simulink model "asbAUV"  (R2024b)
settings: Solver=VariableStepAuto  StartTime=0.0  StopTime=300  FixedStep=0.5  RelTol=1e-3
InitFcn:
  | mdlWks = get_param(gcs,'ModelWorkspace');
  | a = getVariable(mdlWks,'a');
  | b = getVariable(mdlWks,'b');
  | c = getVariable(mdlWks,'c');
StopFcn:
  | fTraj = findobj("Tag","asbAUVTrajectory");
  | 
  | if isempty(fTraj)
  |    fTraj = figure("Tag","asbAUVTrajectory");
  |    axes(fTraj);
  | end
  | 
  | axTraj= gca(fTraj);
  | 
  | if exist('PositionData', 'var')
  |    plot3(axTraj,PositionData(1,1),PositionData(1,2),PositionData(1,3),'r*')
  |    hold on
  |    plot3(axTraj,PositionData(:,1),PositionData(:,2),PositionData(:,3));
  |    plot3(axTraj,PositionData(end,1),PositionData(end,2),PositionData(end,3),'g*');
  | 
  |    axTraj.XLim = [0 15];
  |    axTraj.YLim = [-10 2];
  |    axTraj.ZLim = [-2 12];
  |    axTraj.XLabel.String = 'X (m)';
  |    axTraj.YLabel.String = 'Y (m)';
  |    axTraj.ZLabel.String = 'Z (m)';
  |    grid on
  |    hold off
  | 
  |    legend(axTraj,{'Start Point','Trajectory','End Point'});
  | end
model workspace (MAT data in the model file):
  a = 1
  b = 0
  c = 0
libraries: asbAUVlib x29, dspfdesign x6, slpidlib x6, shared6dof x1, aerolibasang x1, sharedutil x1, aerolibnav x1, SignalEditorBlockLib x1
(part 2 of 3)

== system asbAUV/Plant and Environment Model ==
  Thrust Control : Inport
  Combine Forces and Moments : Subsystem
  Dynamics solver : Subsystem
  Environmental Forces & Moments : Subsystem
  Propulsion Forces & Moments : Subsystem
  Outport : Outport  VectorParamsAs1DForOutWhenUnconnected=off
  wires:
  Thrust Control/1 -> Propulsion Forces & Moments/1(Thrust Control In)
  Propulsion Forces & Moments/1(Propulsion Parameters) -> Combine Forces and Moments/1(Propulsion Parameters)
  Environmental Forces & Moments/1(Environment Parameters) -> Combine Forces and Moments/2(Hydrodynamic Force)
  Combine Forces and Moments/1(Total Force) -> Dynamics solver/1(Total Force)
  Combine Forces and Moments/2(Total Moment) -> Dynamics solver/2(Total Moment)
  Dynamics solver/1(AUV Data) -> Outport/1
  Dynamics solver/2(Internal Parameters) -> Environmental Forces & Moments/1(AOA_SideSlip)

== system asbAUV/Sensor data and State Estimation ==
  AUV_Parameters : Inport
  System With Noise : Subsystem  VariantControl=c==0
  System without Noise : Subsystem  VariantControl=c==1
  Filtered Parameters : Outport  VectorParamsAs1DForOutWhenUnconnected=off

== system asbAUV/Switch Parameters ==
  Constant : Constant  Value=a
  Constant1 : Constant  Value=b
  Constant2 : Constant  Value=c
  Terminator1 : Terminator
  Terminator2 : Terminator
  Terminator3 : Terminator
  wires:
  Constant/1 -> Terminator1/1
  Constant1/1 -> Terminator2/1
  Constant2/1 -> Terminator3/1

== system asbAUV/Translation Controller ==
  Actual Parameters : Inport
  Reference Parameters : Inport  Port=2
  Position Controller : Subsystem  VariantControl=a==0
  Velocity Controller : Subsystem  VariantControl=a==1
  Thrust Control : Outport  VectorParamsAs1DForOutWhenUnconnected=off

== system asbAUV/Translational Reference ==
  Bus Creator : BusCreator  Inputs=2
  Signal Editor : SignalEditorBlockLib/Signal Editor  FileName=asbTransRefScenario.mat  ActiveScenario=asbTransrefScenario  ActiveSignal=Reference Velocity  IsBus=off  OutputBusObjectStr=Bus: BusObject  SampleTime=0  Interpolate=off  ZeroCross=off  OutputAfterFinalValue=Holding final value  Unit=inherit  PreserveSignalName=on  ApplySigPropsToAllScenarios=on  ApplySigPropsToAllSignals=off
  Reference Parameters : Outport  VectorParamsAs1DForOutWhenUnconnected=off
  wires:
  Signal Editor/1 -> Bus Creator/1  "Reference Position"
  Signal Editor/2 -> Bus Creator/2  "Reference Velocity"
  Bus Creator/1 -> Reference Parameters/1

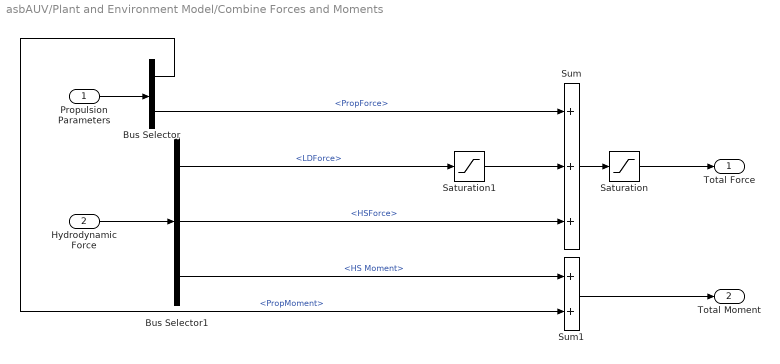
== system asbAUV/Plant and Environment Model/Combine Forces and Moments ==
  Propulsion Parameters : Inport
  Hydrodynamic Force : Inport  Port=2
  Bus Selector : BusSelector  OutputSignals=PropMoment,PropForce
  Bus Selector1 : BusSelector  OutputSignals=LDForce,HSForce,HS Moment
  Saturation : Saturate  UpperLimit=600  LowerLimit=-600
  Saturation1 : Saturate  UpperLimit=600  LowerLimit=-600
  Sum : Sum  Inputs=+++
  Sum1 : Sum
  Total Force : Outport  VectorParamsAs1DForOutWhenUnconnected=off
  Total Moment : Outport  Port=2  VectorParamsAs1DForOutWhenUnconnected=off
  wires:
  Bus Selector1/3 -> Sum1/1  "<HS Moment>"
  Bus Selector/1 -> Sum1/2  "<PropMoment>"
  Sum/1 -> Saturation/1
  Sum1/1 -> Total Moment/1
  Saturation1/1 -> Sum/2
  Saturation/1 -> Total Force/1
  Propulsion Parameters/1 -> Bus Selector/1
  Hydrodynamic Force/1 -> Bus Selector1/1
  Bus Selector/2 -> Sum/1  "<PropForce>"
  Bus Selector1/1 -> Saturation1/1  "<LDForce>"
  Bus Selector1/2 -> Sum/3  "<HSForce>"

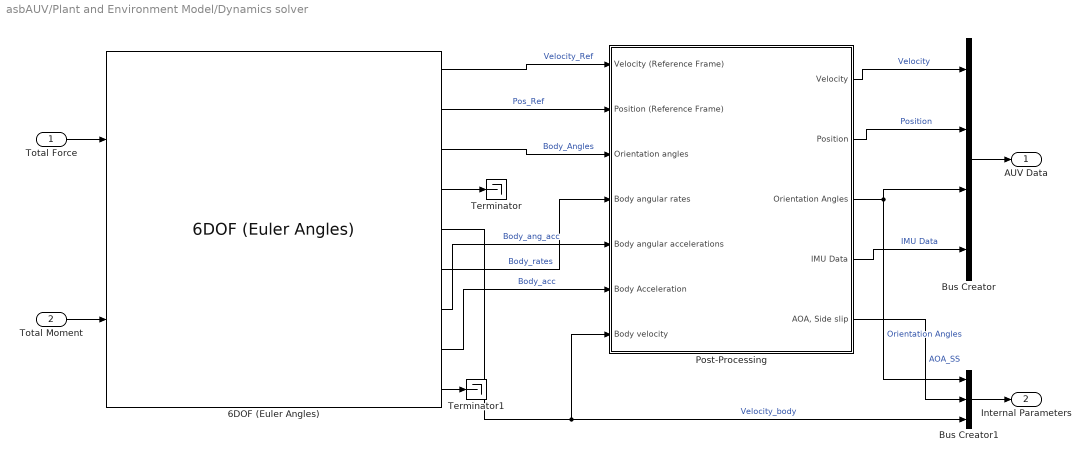
== system asbAUV/Plant and Environment Model/Dynamics solver ==
  Total Force : Inport
  Total Moment : Inport  Port=2
  6DOF (Euler Angles) : shared6dof/6DOF (Euler Angles)  units=Metric (MKS)  mtype=Fixed  rep=Euler Angles  xme_0=[0.01 .01 .01]  Vm_0=[0.01 0.01 0.001]  eul_0=[0.001 0.001 0.001]  pm_0=[0.001 0.001 0.001]  mass_0=10  mass_e=0.5  mass_f=2.0  inertia=10*eye(3)  inertia_e=eye(3)  inertia_f=2*eye(3)  k_quat=1.0  vre_flag=on  abi_flag=on  aMode=0  xme_statename=''  Vm_statename=''  eul_statename=''  quat_statename=''  pm_statename=''  mass_statename=''
  Bus Creator : BusCreator  Inputs=4
  Bus Creator1 : BusCreator  Inputs=3
  Post-Processing : Subsystem
  Terminator : Terminator
  Terminator1 : Terminator
  AUV Data : Outport  VectorParamsAs1DForOutWhenUnconnected=off
  Internal Parameters : Outport  Port=2  VectorParamsAs1DForOutWhenUnconnected=off
  wires:
  6DOF (Euler Angles)/6 -> Post-Processing/4(Body angular rates)  "Body_rates"
  Post-Processing/5("AOA, Side slip") -> Bus Creator1/2  "AOA_SS"
  6DOF (Euler Angles)/8 -> Post-Processing/6(Body Acceleration)  "Body_acc"
  Post-Processing/2(" Position") -> Bus Creator/2  "Position"
  6DOF (Euler Angles)/7 -> Post-Processing/5(Body angular accelerations)  "Body_ang_acc"
  6DOF (Euler Angles)/2 -> Post-Processing/2(Position (Reference Frame))  "Pos_Ref"
  6DOF (Euler Angles)/3 -> Post-Processing/3(Orientation angles)  "Body_Angles"
  Post-Processing/1(Velocity) -> Bus Creator/1  "Velocity"
  6DOF (Euler Angles)/1 -> Post-Processing/1(Velocity (Reference Frame))  "Velocity_Ref"
  6DOF (Euler Angles)/5 -> Bus Creator1/3, Post-Processing/7(Body velocity)  "Velocity_body"
  Post-Processing/3(Orientation Angles) -> Bus Creator/3, Bus Creator1/1  "Orientation Angles"
  Post-Processing/4(IMU Data) -> Bus Creator/4  "IMU Data"
  Total Force/1 -> 6DOF (Euler Angles)/1
  Total Moment/1 -> 6DOF (Euler Angles)/2
  Bus Creator/1 -> AUV Data/1
  Bus Creator1/1 -> Internal Parameters/1
  6DOF (Euler Angles)/4 -> Terminator/1
  6DOF (Euler Angles)/9 -> Terminator1/1

== system asbAUV/Plant and Environment Model/Environmental Forces & Moments ==
  AOA_SideSlip : Inport
  Bus Creator : BusCreator  Inputs=3
  Bus Selector : BusSelector  OutputSignals=Velocity_body,AOA_SS,Orientation Angles
  Hydrodynamic Forces : Subsystem  Variant=on
  Hydrostatic Forces : Subsystem
  Environment Parameters : Outport  VectorParamsAs1DForOutWhenUnconnected=off
  wires:
  Hydrodynamic Forces/1("Force due to Lift, Drag") -> Bus Creator/1  "LDForce"
  Hydrostatic Forces/1(Hydrostatic Force) -> Bus Creator/2  "HSForce"
  Hydrostatic Forces/2(Hydrostatic Moment) -> Bus Creator/3  "HS Moment"
  Bus Creator/1 -> Environment Parameters/1
  AOA_SideSlip/1 -> Bus Selector/1
  Bus Selector/1 -> Hydrodynamic Forces/1("Submarine Velocity (Body Axis) ")  "<Velocity_body>"
  Bus Selector/2 -> Hydrodynamic Forces/2("AOA, Side Slip")  "<AOA_SS>"
  Bus Selector/3 -> Hydrostatic Forces/1(In1)  "<Orientation Angles>"

== system asbAUV/Plant and Environment Model/Propulsion Forces & Moments ==
  Thrust Control In : Inport
  Bus Creator : BusCreator  Inputs=2
  Force and moments due to Thrust : Subsystem
  Input commands to Thrust : Subsystem
  Propulsion Parameters : Outport  VectorParamsAs1DForOutWhenUnconnected=off
  wires:
  Input commands to Thrust/1(Thrust values) -> Force and moments due to Thrust/1(Thrust Inputs)
  Thrust Control In/1 -> Input commands to Thrust/1(Thrust Control Inputs)
  Force and moments due to Thrust/1(Propulsion Force) -> Bus Creator/1  "PropForce"
  Force and moments due to Thrust/2(Propulsion Moment) -> Bus Creator/2  "PropMoment"
  Bus Creator/1 -> Propulsion Parameters/1

== system asbAUV/Sensor data and State Estimation/System With Noise ==
  AUV_Parameters : Inport
  " Sensor (IMU)" : Subsystem
  Internal filter : Subsystem
  Filtered Parameters : Outport  VectorParamsAs1DForOutWhenUnconnected=off
  wires:
  AUV_Parameters/1 -> " Sensor (IMU)"/1(IMU Inputs)
  Internal filter/1(Filtered Parameters) -> Filtered Parameters/1
  " Sensor (IMU)"/1(IMU Measurements) -> Internal filter/1(Accel)

== system asbAUV/Sensor data and State Estimation/System without Noise ==
  AUV_Parameters : Inport
  Bus Creator : BusCreator  Inputs=2
  Bus Selector : BusSelector  OutputSignals=Position,Velocity
  Gain : Gain
  Gain1 : Gain
  Filtered Parameters : Outport  VectorParamsAs1DForOutWhenUnconnected=off
  wires:
  Bus Creator/1 -> Filtered Parameters/1
  Bus Selector/2 -> Gain1/1  "<Velocity>"
  Bus Selector/1 -> Gain/1  "<Position>"
  Gain1/1 -> Bus Creator/2  "Filtered Velocity"
  Gain/1 -> Bus Creator/1  "Filtered Position"
  AUV_Parameters/1 -> Bus Selector/1

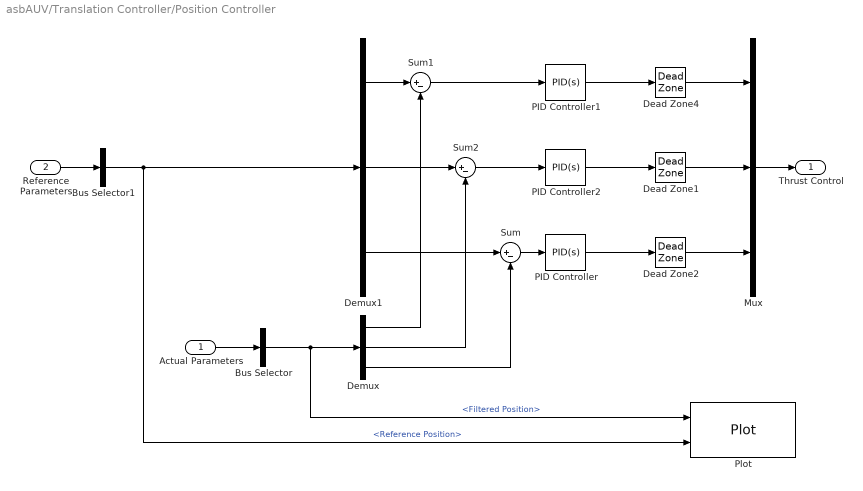
== system asbAUV/Translation Controller/Position Controller ==
  Actual Parameters : Inport
  Reference Parameters : Inport  Port=2
  Bus Selector : BusSelector  OutputSignals=Filtered Position
  Bus Selector1 : BusSelector  OutputSignals=Reference Position
  Dead Zone1 : DeadZone  LowerValue=-0.05  UpperValue=+0.05
  Dead Zone2 : DeadZone  LowerValue=-0.05  UpperValue=+0.05
  Dead Zone4 : DeadZone  LowerValue=-0.05  UpperValue=+0.05
  Demux : Demux  Outputs=3
  Demux1 : Demux  Outputs=3
  Mux : Mux  Inputs=3
  PID Controller : slpidlib/PID Controller  Controller=PID  Form=Parallel  TimeDomain=Continuous-time  UseExternalTs=off  SampleTime=-1  IntegratorMethod=Forward Euler  FilterMethod=Forward Euler  ControllerParametersSource=internal  P=-0.0440831016133051  I=-0.00046335965727533  UseKiTs=off  D=-0.931852208113014  UseExternalDerivativeSource=off  N=205.904485551143  UseFilter=on  TunerSelectOption=Transfer Function Based (PID Tuner App)  InitialConditionSource=internal  InitialConditionForIntegrator=0  InitialConditionForFilter=0  DifferentiatorICPrevScaledInput=0  ExternalReset=none  TrackingMode=off  Kt=1  LimitOutput=off  SatLimitsSource=internal  UpperSaturationLimit=inf  LowerSaturationLimit=-inf  LinearizeAsGain=on  AntiWindupMode=none  Kb=1  LimitIntegrator=off  UpperIntegratorSaturationLimit=inf  LowerIntegratorSaturationLimit=-inf  POutMin=[]  POutMax=[]  IOutMin=[]  IOutMax=[]  DOutMin=[]  DOutMax=[]  NOutMin=[]  NOutMax=[]  SumOutMin=[]  SumOutMax=[]  SaturationOutMin=[]  SaturationOutMax=[]  PParamMin=[]  PParamMax=[]  IParamMin=[]  IParamMax=[]  DParamMin=[]  DParamMax=[]  NParamMin=[]  NParamMax=[]  KbParamMin=[]  KbParamMax=[]  KtParamMin=[]  KtParamMax=[]  KbOutMin=[]  KbOutMax=[]  KtOutMin=[]  KtOutMax=[]  IntegratorOutMin=[]  IntegratorOutMax=[]  FilterOutMin=[]  FilterOutMax=[]  SumI1OutMin=[]  SumI1OutMax=[]  SumI2OutMin=[]  SumI2OutMax=[]  SumI3OutMin=[]  SumI3OutMax=[]  SumI4OutMin=[]  SumI4OutMax=[]  SumDOutMin=[]  SumDOutMax=[]  DifferentiatorOutMin=[]  DifferentiatorOutMax=[]  FilterDiffOutCoefMin=[]  FilterDiffOutCoefMax=[]  ReciprocalOutMin=[]  ReciprocalOutMax=[]  SumDenOutMin=[]  SumDenOutMax=[]  SumNumOutMin=[]  SumNumOutMax=[]  DivideOutMin=[]  DivideOutMax=[]  UdiffTsProdOutMin=[]  UdiffTsProdOutMax=[]  NTsProdOutMin=[]  NTsProdOutMax=[]  UintegralTsProdOutMin=[]  UintegralTsProdOutMax=[]  UngainTsProdOutMin=[]  UngainTsProdOutMax=[]  ClampingZeroOutDataTypeStr=Inherit: Inherit via back propagation  ClampingZeroOutMin=[]  ClampingZeroOutMax=[]  FilterDenConstantOutDataTypeStr=Inherit: Inherit via back propagation  FilterDenConstantOutMin=[]  FilterDenConstantOutMax=[]  PCopyOutDataTypeStr=Inherit: Inherit via back propagation  PCopyOutMin=[]  PCopyOutMax=[]  NCopyOutDataTypeStr=Inherit: Inherit via back propagation  NCopyOutMin=[]  NCopyOutMax=[]  IntegratorContinuousStateAttributes=''  IntegratorStateMustResolveToSignalObject=off  IntegratorRTWStateStorageClass=Auto  FilterContinuousStateAttributes=''  FilterStateMustResolveToSignalObject=off  FilterRTWStateStorageClass=Auto  ParallelPVariant=InternalParameters  IdealPVariant=Disabled  IVariant=InternalParameters  DVariant=InternalParameters  IntegratorVariant=Continuous  SatVariant=Disabled  AWVariant=Passthrough  PCopyVariant=Disabled  TRVariant=Disabled  FdbkBlocksVariant=Forward  IdealPFdbkVariant=Disabled  SatFdbkVariant=Disabled  DerivativeFilterVariant=ContFilter  NVariant=InternalParameters  NCopyVariant=Disabled  FilterICVariant=InternalICsFilter  IntegratorICVariant=InternalICs  ExternalResetVariant=Disabled  TRSumVariant=Passthrough  SumFdbkVariant=Disabled  SumVariant=Sum_PID  TsampFilterVariant=InternalTs  TsampNgainVariant=Passthrough  TsampIntegralVariant=Disabled_SignalSpec  ExternalSaturationOutDataTypeStr=Inherit: Same as second input  DerivativeSourceVariant=ErrorSignal  PreIntVariant=InternalPreInt
  PID Controller1 : slpidlib/PID Controller  Controller=PID  Form=Parallel  TimeDomain=Continuous-time  UseExternalTs=off  SampleTime=-1  IntegratorMethod=Forward Euler  FilterMethod=Forward Euler  ControllerParametersSource=internal  P=0.0352909553215239  I=0.000468513300704798  UseKiTs=off  D=0.59064410837381  UseExternalDerivativeSource=off  N=260.062804539004  UseFilter=on  TunerSelectOption=Transfer Function Based (PID Tuner App)  InitialConditionSource=internal  InitialConditionForIntegrator=0  InitialConditionForFilter=0  DifferentiatorICPrevScaledInput=0  ExternalReset=none  TrackingMode=off  Kt=1  LimitOutput=off  SatLimitsSource=internal  UpperSaturationLimit=inf  LowerSaturationLimit=-inf  LinearizeAsGain=on  AntiWindupMode=none  Kb=1  LimitIntegrator=off  UpperIntegratorSaturationLimit=inf  LowerIntegratorSaturationLimit=-inf  POutMin=[]  POutMax=[]  IOutMin=[]  IOutMax=[]  DOutMin=[]  DOutMax=[]  NOutMin=[]  NOutMax=[]  SumOutMin=[]  SumOutMax=[]  SaturationOutMin=[]  SaturationOutMax=[]  PParamMin=[]  PParamMax=[]  IParamMin=[]  IParamMax=[]  DParamMin=[]  DParamMax=[]  NParamMin=[]  NParamMax=[]  KbParamMin=[]  KbParamMax=[]  KtParamMin=[]  KtParamMax=[]  KbOutMin=[]  KbOutMax=[]  KtOutMin=[]  KtOutMax=[]  IntegratorOutMin=[]  IntegratorOutMax=[]  FilterOutMin=[]  FilterOutMax=[]  SumI1OutMin=[]  SumI1OutMax=[]  SumI2OutMin=[]  SumI2OutMax=[]  SumI3OutMin=[]  SumI3OutMax=[]  SumI4OutMin=[]  SumI4OutMax=[]  SumDOutMin=[]  SumDOutMax=[]  DifferentiatorOutMin=[]  DifferentiatorOutMax=[]  FilterDiffOutCoefMin=[]  FilterDiffOutCoefMax=[]  ReciprocalOutMin=[]  ReciprocalOutMax=[]  SumDenOutMin=[]  SumDenOutMax=[]  SumNumOutMin=[]  SumNumOutMax=[]  DivideOutMin=[]  DivideOutMax=[]  UdiffTsProdOutMin=[]  UdiffTsProdOutMax=[]  NTsProdOutMin=[]  NTsProdOutMax=[]  UintegralTsProdOutMin=[]  UintegralTsProdOutMax=[]  UngainTsProdOutMin=[]  UngainTsProdOutMax=[]  ClampingZeroOutDataTypeStr=Inherit: Inherit via back propagation  ClampingZeroOutMin=[]  ClampingZeroOutMax=[]  FilterDenConstantOutDataTypeStr=Inherit: Inherit via back propagation  FilterDenConstantOutMin=[]  FilterDenConstantOutMax=[]  PCopyOutDataTypeStr=Inherit: Inherit via back propagation  PCopyOutMin=[]  PCopyOutMax=[]  NCopyOutDataTypeStr=Inherit: Inherit via back propagation  NCopyOutMin=[]  NCopyOutMax=[]  IntegratorContinuousStateAttributes=''  IntegratorStateMustResolveToSignalObject=off  IntegratorRTWStateStorageClass=Auto  FilterContinuousStateAttributes=''  FilterStateMustResolveToSignalObject=off  FilterRTWStateStorageClass=Auto  ParallelPVariant=InternalParameters  IdealPVariant=Disabled  IVariant=InternalParameters  DVariant=InternalParameters  IntegratorVariant=Continuous  SatVariant=Disabled  AWVariant=Passthrough  PCopyVariant=Disabled  TRVariant=Disabled  FdbkBlocksVariant=Forward  IdealPFdbkVariant=Disabled  SatFdbkVariant=Disabled  DerivativeFilterVariant=ContFilter  NVariant=InternalParameters  NCopyVariant=Disabled  FilterICVariant=InternalICsFilter  IntegratorICVariant=InternalICs  ExternalResetVariant=Disabled  TRSumVariant=Passthrough  SumFdbkVariant=Disabled  SumVariant=Sum_PID  TsampFilterVariant=InternalTs  TsampNgainVariant=Passthrough  TsampIntegralVariant=Disabled_SignalSpec  ExternalSaturationOutDataTypeStr=Inherit: Same as second input  DerivativeSourceVariant=ErrorSignal  PreIntVariant=InternalPreInt
  PID Controller2 : slpidlib/PID Controller  Controller=PID  Form=Parallel  TimeDomain=Continuous-time  UseExternalTs=off  SampleTime=-1  IntegratorMethod=Forward Euler  FilterMethod=Forward Euler  ControllerParametersSource=internal  P=0.172975950646219  I=0.00387308418128247  UseKiTs=off  D=1.71646711354372  UseExternalDerivativeSource=off  N=438.622536688858  UseFilter=on  TunerSelectOption=Transfer Function Based (PID Tuner App)  InitialConditionSource=internal  InitialConditionForIntegrator=0  InitialConditionForFilter=0  DifferentiatorICPrevScaledInput=0  ExternalReset=none  TrackingMode=off  Kt=1  LimitOutput=off  SatLimitsSource=internal  UpperSaturationLimit=inf  LowerSaturationLimit=-inf  LinearizeAsGain=on  AntiWindupMode=none  Kb=1  LimitIntegrator=off  UpperIntegratorSaturationLimit=inf  LowerIntegratorSaturationLimit=-inf  POutMin=[]  POutMax=[]  IOutMin=[]  IOutMax=[]  DOutMin=[]  DOutMax=[]  NOutMin=[]  NOutMax=[]  SumOutMin=[]  SumOutMax=[]  SaturationOutMin=[]  SaturationOutMax=[]  PParamMin=[]  PParamMax=[]  IParamMin=[]  IParamMax=[]  DParamMin=[]  DParamMax=[]  NParamMin=[]  NParamMax=[]  KbParamMin=[]  KbParamMax=[]  KtParamMin=[]  KtParamMax=[]  KbOutMin=[]  KbOutMax=[]  KtOutMin=[]  KtOutMax=[]  IntegratorOutMin=[]  IntegratorOutMax=[]  FilterOutMin=[]  FilterOutMax=[]  SumI1OutMin=[]  SumI1OutMax=[]  SumI2OutMin=[]  SumI2OutMax=[]  SumI3OutMin=[]  SumI3OutMax=[]  SumI4OutMin=[]  SumI4OutMax=[]  SumDOutMin=[]  SumDOutMax=[]  DifferentiatorOutMin=[]  DifferentiatorOutMax=[]  FilterDiffOutCoefMin=[]  FilterDiffOutCoefMax=[]  ReciprocalOutMin=[]  ReciprocalOutMax=[]  SumDenOutMin=[]  SumDenOutMax=[]  SumNumOutMin=[]  SumNumOutMax=[]  DivideOutMin=[]  DivideOutMax=[]  UdiffTsProdOutMin=[]  UdiffTsProdOutMax=[]  NTsProdOutMin=[]  NTsProdOutMax=[]  UintegralTsProdOutMin=[]  UintegralTsProdOutMax=[]  UngainTsProdOutMin=[]  UngainTsProdOutMax=[]  ClampingZeroOutDataTypeStr=Inherit: Inherit via back propagation  ClampingZeroOutMin=[]  ClampingZeroOutMax=[]  FilterDenConstantOutDataTypeStr=Inherit: Inherit via back propagation  FilterDenConstantOutMin=[]  FilterDenConstantOutMax=[]  PCopyOutDataTypeStr=Inherit: Inherit via back propagation  PCopyOutMin=[]  PCopyOutMax=[]  NCopyOutDataTypeStr=Inherit: Inherit via back propagation  NCopyOutMin=[]  NCopyOutMax=[]  IntegratorContinuousStateAttributes=''  IntegratorStateMustResolveToSignalObject=off  IntegratorRTWStateStorageClass=Auto  FilterContinuousStateAttributes=''  FilterStateMustResolveToSignalObject=off  FilterRTWStateStorageClass=Auto  ParallelPVariant=InternalParameters  IdealPVariant=Disabled  IVariant=InternalParameters  DVariant=InternalParameters  IntegratorVariant=Continuous  SatVariant=Disabled  AWVariant=Passthrough  PCopyVariant=Disabled  TRVariant=Disabled  FdbkBlocksVariant=Forward  IdealPFdbkVariant=Disabled  SatFdbkVariant=Disabled  DerivativeFilterVariant=ContFilter  NVariant=InternalParameters  NCopyVariant=Disabled  FilterICVariant=InternalICsFilter  IntegratorICVariant=InternalICs  ExternalResetVariant=Disabled  TRSumVariant=Passthrough  SumFdbkVariant=Disabled  SumVariant=Sum_PID  TsampFilterVariant=InternalTs  TsampNgainVariant=Passthrough  TsampIntegralVariant=Disabled_SignalSpec  ExternalSaturationOutDataTypeStr=Inherit: Same as second input  DerivativeSourceVariant=ErrorSignal  PreIntVariant=InternalPreInt
  Plot : asbAUVlib/Plot  SystemSampleTime=-1  VariantActivationTime=update diagram  AllowFlexibleInterface=on  Latency=0  AutoFrameSizeCalculation=off
  Sum : Sum  Inputs=|+-
  Sum1 : Sum  Inputs=|+-
  Sum2 : Sum  Inputs=|+-
  Thrust Control : Outport  VectorParamsAs1DForOutWhenUnconnected=off
  wires:
  Demux1/1 -> Sum1/1
  Demux1/3 -> Sum/1
  Demux1/2 -> Sum2/1
  PID Controller1/1 -> Dead Zone4/1
  Demux/3 -> Sum/2
  PID Controller2/1 -> Dead Zone1/1
  Demux/2 -> Sum2/2
  Sum2/1 -> PID Controller2/1
  Demux/1 -> Sum1/2
  Sum/1 -> PID Controller/1
  PID Controller/1 -> Dead Zone2/1
  Sum1/1 -> PID Controller1/1
  Mux/1 -> Thrust Control/1
  Dead Zone4/1 -> Mux/1
  Dead Zone1/1 -> Mux/2
  Dead Zone2/1 -> Mux/3
  Actual Parameters/1 -> Bus Selector/1
  Bus Selector/1 -> Plot/1, Demux/1  "<Filtered Position>"
  Reference Parameters/1 -> Bus Selector1/1
  Bus Selector1/1 -> Plot/2, Demux1/1  "<Reference Position>"

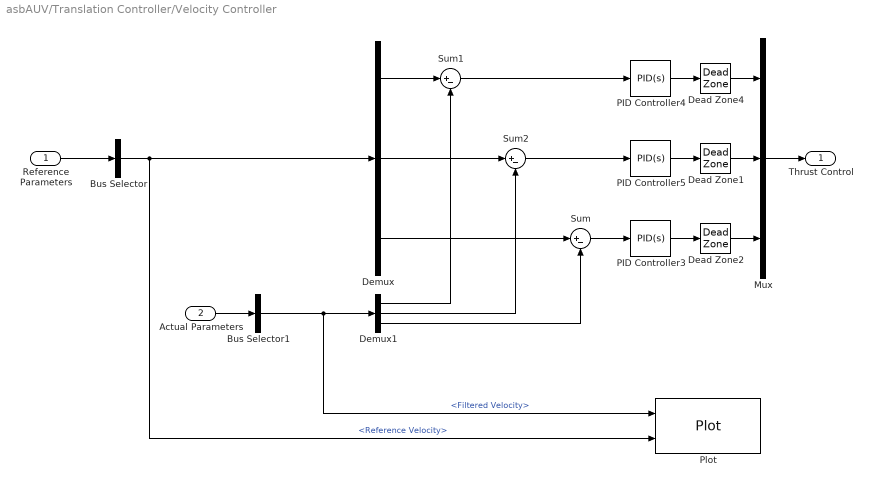
== system asbAUV/Translation Controller/Velocity Controller ==
  Reference Parameters : Inport
  Actual Parameters : Inport  Port=2
  Bus Selector : BusSelector  OutputSignals=Reference Velocity
  Bus Selector1 : BusSelector  OutputSignals=Filtered Velocity
  Dead Zone1 : DeadZone  LowerValue=-0.05  UpperValue=+0.05
  Dead Zone2 : DeadZone  LowerValue=-0.05  UpperValue=+0.05
  Dead Zone4 : DeadZone  LowerValue=-0.05  UpperValue=+0.05
  Demux : Demux  Outputs=3
  Demux1 : Demux  Outputs=3
  Mux : Mux  Inputs=3
  PID Controller3 : slpidlib/PID Controller  Controller=PID  Form=Parallel  TimeDomain=Continuous-time  UseExternalTs=off  SampleTime=-1  IntegratorMethod=Forward Euler  FilterMethod=Forward Euler  ControllerParametersSource=internal  P=-0.61964554396314  I=-0.140214385843897  UseKiTs=off  D=0.00440045709674139  UseExternalDerivativeSource=off  N=140.813904178727  UseFilter=on  TunerSelectOption=Transfer Function Based (PID Tuner App)  InitialConditionSource=internal  InitialConditionForIntegrator=0  InitialConditionForFilter=0  DifferentiatorICPrevScaledInput=0  ExternalReset=none  TrackingMode=off  Kt=1  LimitOutput=off  SatLimitsSource=internal  UpperSaturationLimit=inf  LowerSaturationLimit=-inf  LinearizeAsGain=on  AntiWindupMode=none  Kb=1  LimitIntegrator=off  UpperIntegratorSaturationLimit=inf  LowerIntegratorSaturationLimit=-inf  POutMin=[]  POutMax=[]  IOutMin=[]  IOutMax=[]  DOutMin=[]  DOutMax=[]  NOutMin=[]  NOutMax=[]  SumOutMin=[]  SumOutMax=[]  SaturationOutMin=[]  SaturationOutMax=[]  PParamMin=[]  PParamMax=[]  IParamMin=[]  IParamMax=[]  DParamMin=[]  DParamMax=[]  NParamMin=[]  NParamMax=[]  KbParamMin=[]  KbParamMax=[]  KtParamMin=[]  KtParamMax=[]  KbOutMin=[]  KbOutMax=[]  KtOutMin=[]  KtOutMax=[]  IntegratorOutMin=[]  IntegratorOutMax=[]  FilterOutMin=[]  FilterOutMax=[]  SumI1OutMin=[]  SumI1OutMax=[]  SumI2OutMin=[]  SumI2OutMax=[]  SumI3OutMin=[]  SumI3OutMax=[]  SumI4OutMin=[]  SumI4OutMax=[]  SumDOutMin=[]  SumDOutMax=[]  DifferentiatorOutMin=[]  DifferentiatorOutMax=[]  FilterDiffOutCoefMin=[]  FilterDiffOutCoefMax=[]  ReciprocalOutMin=[]  ReciprocalOutMax=[]  SumDenOutMin=[]  SumDenOutMax=[]  SumNumOutMin=[]  SumNumOutMax=[]  DivideOutMin=[]  DivideOutMax=[]  UdiffTsProdOutMin=[]  UdiffTsProdOutMax=[]  NTsProdOutMin=[]  NTsProdOutMax=[]  UintegralTsProdOutMin=[]  UintegralTsProdOutMax=[]  UngainTsProdOutMin=[]  UngainTsProdOutMax=[]  ClampingZeroOutDataTypeStr=Inherit: Inherit via back propagation  ClampingZeroOutMin=[]  ClampingZeroOutMax=[]  FilterDenConstantOutDataTypeStr=Inherit: Inherit via back propagation  FilterDenConstantOutMin=[]  FilterDenConstantOutMax=[]  PCopyOutDataTypeStr=Inherit: Inherit via back propagation  PCopyOutMin=[]  PCopyOutMax=[]  NCopyOutDataTypeStr=Inherit: Inherit via back propagation  NCopyOutMin=[]  NCopyOutMax=[]  IntegratorContinuousStateAttributes=''  IntegratorStateMustResolveToSignalObject=off  IntegratorRTWStateStorageClass=Auto  FilterContinuousStateAttributes=''  FilterStateMustResolveToSignalObject=off  FilterRTWStateStorageClass=Auto  ParallelPVariant=InternalParameters  IdealPVariant=Disabled  IVariant=InternalParameters  DVariant=InternalParameters  IntegratorVariant=Continuous  SatVariant=Disabled  AWVariant=Passthrough  PCopyVariant=Disabled  TRVariant=Disabled  FdbkBlocksVariant=Forward  IdealPFdbkVariant=Disabled  SatFdbkVariant=Disabled  DerivativeFilterVariant=ContFilter  NVariant=InternalParameters  NCopyVariant=Disabled  FilterICVariant=InternalICsFilter  IntegratorICVariant=InternalICs  ExternalResetVariant=Disabled  TRSumVariant=Passthrough  SumFdbkVariant=Disabled  SumVariant=Sum_PID  TsampFilterVariant=InternalTs  TsampNgainVariant=Passthrough  TsampIntegralVariant=Disabled_SignalSpec  ExternalSaturationOutDataTypeStr=Inherit: Same as second input  DerivativeSourceVariant=ErrorSignal  PreIntVariant=InternalPreInt
  PID Controller4 : slpidlib/PID Controller  Controller=PID  Form=Parallel  TimeDomain=Continuous-time  UseExternalTs=off  SampleTime=-1  IntegratorMethod=Forward Euler  FilterMethod=Forward Euler  ControllerParametersSource=internal  P=0.262050505979025  I=0.0518732197045156  UseKiTs=off  D=-0.0235509594288088  UseExternalDerivativeSource=off  N=11.1269567072699  UseFilter=on  TunerSelectOption=Transfer Function Based (PID Tuner App)  InitialConditionSource=internal  InitialConditionForIntegrator=0  InitialConditionForFilter=0  DifferentiatorICPrevScaledInput=0  ExternalReset=none  TrackingMode=off  Kt=1  LimitOutput=off  SatLimitsSource=internal  UpperSaturationLimit=inf  LowerSaturationLimit=-inf  LinearizeAsGain=on  AntiWindupMode=none  Kb=1  LimitIntegrator=off  UpperIntegratorSaturationLimit=inf  LowerIntegratorSaturationLimit=-inf  POutMin=[]  POutMax=[]  IOutMin=[]  IOutMax=[]  DOutMin=[]  DOutMax=[]  NOutMin=[]  NOutMax=[]  SumOutMin=[]  SumOutMax=[]  SaturationOutMin=[]  SaturationOutMax=[]  PParamMin=[]  PParamMax=[]  IParamMin=[]  IParamMax=[]  DParamMin=[]  DParamMax=[]  NParamMin=[]  NParamMax=[]  KbParamMin=[]  KbParamMax=[]  KtParamMin=[]  KtParamMax=[]  KbOutMin=[]  KbOutMax=[]  KtOutMin=[]  KtOutMax=[]  IntegratorOutMin=[]  IntegratorOutMax=[]  FilterOutMin=[]  FilterOutMax=[]  SumI1OutMin=[]  SumI1OutMax=[]  SumI2OutMin=[]  SumI2OutMax=[]  SumI3OutMin=[]  SumI3OutMax=[]  SumI4OutMin=[]  SumI4OutMax=[]  SumDOutMin=[]  SumDOutMax=[]  DifferentiatorOutMin=[]  DifferentiatorOutMax=[]  FilterDiffOutCoefMin=[]  FilterDiffOutCoefMax=[]  ReciprocalOutMin=[]  ReciprocalOutMax=[]  SumDenOutMin=[]  SumDenOutMax=[]  SumNumOutMin=[]  SumNumOutMax=[]  DivideOutMin=[]  DivideOutMax=[]  UdiffTsProdOutMin=[]  UdiffTsProdOutMax=[]  NTsProdOutMin=[]  NTsProdOutMax=[]  UintegralTsProdOutMin=[]  UintegralTsProdOutMax=[]  UngainTsProdOutMin=[]  UngainTsProdOutMax=[]  ClampingZeroOutDataTypeStr=Inherit: Inherit via back propagation  ClampingZeroOutMin=[]  ClampingZeroOutMax=[]  FilterDenConstantOutDataTypeStr=Inherit: Inherit via back propagation  FilterDenConstantOutMin=[]  FilterDenConstantOutMax=[]  PCopyOutDataTypeStr=Inherit: Inherit via back propagation  PCopyOutMin=[]  PCopyOutMax=[]  NCopyOutDataTypeStr=Inherit: Inherit via back propagation  NCopyOutMin=[]  NCopyOutMax=[]  IntegratorContinuousStateAttributes=''  IntegratorStateMustResolveToSignalObject=off  IntegratorRTWStateStorageClass=Auto  FilterContinuousStateAttributes=''  FilterStateMustResolveToSignalObject=off  FilterRTWStateStorageClass=Auto  ParallelPVariant=InternalParameters  IdealPVariant=Disabled  IVariant=InternalParameters  DVariant=InternalParameters  IntegratorVariant=Continuous  SatVariant=Disabled  AWVariant=Passthrough  PCopyVariant=Disabled  TRVariant=Disabled  FdbkBlocksVariant=Forward  IdealPFdbkVariant=Disabled  SatFdbkVariant=Disabled  DerivativeFilterVariant=ContFilter  NVariant=InternalParameters  NCopyVariant=Disabled  FilterICVariant=InternalICsFilter  IntegratorICVariant=InternalICs  ExternalResetVariant=Disabled  TRSumVariant=Passthrough  SumFdbkVariant=Disabled  SumVariant=Sum_PID  TsampFilterVariant=InternalTs  TsampNgainVariant=Passthrough  TsampIntegralVariant=Disabled_SignalSpec  ExternalSaturationOutDataTypeStr=Inherit: Same as second input  DerivativeSourceVariant=ErrorSignal  PreIntVariant=InternalPreInt
  PID Controller5 : slpidlib/PID Controller  Controller=PID  Form=Parallel  TimeDomain=Continuous-time  UseExternalTs=off  SampleTime=-1  IntegratorMethod=Forward Euler  FilterMethod=Forward Euler  ControllerParametersSource=internal  P=1.14371295451496  I=0.548529610159355  UseKiTs=off  D=-0.00383210771245667  UseExternalDerivativeSource=off  N=298.455325458939  UseFilter=on  TunerSelectOption=Transfer Function Based (PID Tuner App)  InitialConditionSource=internal  InitialConditionForIntegrator=0  InitialConditionForFilter=0  DifferentiatorICPrevScaledInput=0  ExternalReset=none  TrackingMode=off  Kt=1  LimitOutput=off  SatLimitsSource=internal  UpperSaturationLimit=inf  LowerSaturationLimit=-inf  LinearizeAsGain=on  AntiWindupMode=none  Kb=1  LimitIntegrator=off  UpperIntegratorSaturationLimit=inf  LowerIntegratorSaturationLimit=-inf  POutMin=[]  POutMax=[]  IOutMin=[]  IOutMax=[]  DOutMin=[]  DOutMax=[]  NOutMin=[]  NOutMax=[]  SumOutMin=[]  SumOutMax=[]  SaturationOutMin=[]  SaturationOutMax=[]  PParamMin=[]  PParamMax=[]  IParamMin=[]  IParamMax=[]  DParamMin=[]  DParamMax=[]  NParamMin=[]  NParamMax=[]  KbParamMin=[]  KbParamMax=[]  KtParamMin=[]  KtParamMax=[]  KbOutMin=[]  KbOutMax=[]  KtOutMin=[]  KtOutMax=[]  IntegratorOutMin=[]  IntegratorOutMax=[]  FilterOutMin=[]  FilterOutMax=[]  SumI1OutMin=[]  SumI1OutMax=[]  SumI2OutMin=[]  SumI2OutMax=[]  SumI3OutMin=[]  SumI3OutMax=[]  SumI4OutMin=[]  SumI4OutMax=[]  SumDOutMin=[]  SumDOutMax=[]  DifferentiatorOutMin=[]  DifferentiatorOutMax=[]  FilterDiffOutCoefMin=[]  FilterDiffOutCoefMax=[]  ReciprocalOutMin=[]  ReciprocalOutMax=[]  SumDenOutMin=[]  SumDenOutMax=[]  SumNumOutMin=[]  SumNumOutMax=[]  DivideOutMin=[]  DivideOutMax=[]  UdiffTsProdOutMin=[]  UdiffTsProdOutMax=[]  NTsProdOutMin=[]  NTsProdOutMax=[]  UintegralTsProdOutMin=[]  UintegralTsProdOutMax=[]  UngainTsProdOutMin=[]  UngainTsProdOutMax=[]  ClampingZeroOutDataTypeStr=Inherit: Inherit via back propagation  ClampingZeroOutMin=[]  ClampingZeroOutMax=[]  FilterDenConstantOutDataTypeStr=Inherit: Inherit via back propagation  FilterDenConstantOutMin=[]  FilterDenConstantOutMax=[]  PCopyOutDataTypeStr=Inherit: Inherit via back propagation  PCopyOutMin=[]  PCopyOutMax=[]  NCopyOutDataTypeStr=Inherit: Inherit via back propagation  NCopyOutMin=[]  NCopyOutMax=[]  IntegratorContinuousStateAttributes=''  IntegratorStateMustResolveToSignalObject=off  IntegratorRTWStateStorageClass=Auto  FilterContinuousStateAttributes=''  FilterStateMustResolveToSignalObject=off  FilterRTWStateStorageClass=Auto  ParallelPVariant=InternalParameters  IdealPVariant=Disabled  IVariant=InternalParameters  DVariant=InternalParameters  IntegratorVariant=Continuous  SatVariant=Disabled  AWVariant=Passthrough  PCopyVariant=Disabled  TRVariant=Disabled  FdbkBlocksVariant=Forward  IdealPFdbkVariant=Disabled  SatFdbkVariant=Disabled  DerivativeFilterVariant=ContFilter  NVariant=InternalParameters  NCopyVariant=Disabled  FilterICVariant=InternalICsFilter  IntegratorICVariant=InternalICs  ExternalResetVariant=Disabled  TRSumVariant=Passthrough  SumFdbkVariant=Disabled  SumVariant=Sum_PID  TsampFilterVariant=InternalTs  TsampNgainVariant=Passthrough  TsampIntegralVariant=Disabled_SignalSpec  ExternalSaturationOutDataTypeStr=Inherit: Same as second input  DerivativeSourceVariant=ErrorSignal  PreIntVariant=InternalPreInt
  Plot : asbAUVlib/Plot  SystemSampleTime=-1  VariantActivationTime=update diagram  AllowFlexibleInterface=on  Latency=0  AutoFrameSizeCalculation=off
  Sum : Sum  Inputs=|+-
  Sum1 : Sum  Inputs=|+-
  Sum2 : Sum  Inputs=|+-
  Thrust Control : Outport  VectorParamsAs1DForOutWhenUnconnected=off
  wires:
  Demux1/3 -> Sum/2
  PID Controller3/1 -> Dead Zone2/1
  Demux/3 -> Sum/1
  PID Controller4/1 -> Dead Zone4/1
  PID Controller5/1 -> Dead Zone1/1
  Demux/2 -> Sum2/1
  Dead Zone2/1 -> Mux/3
  Dead Zone1/1 -> Mux/2
  Demux/1 -> Sum1/1
  Demux1/1 -> Sum1/2
  Demux1/2 -> Sum2/2
  Dead Zone4/1 -> Mux/1
  Mux/1 -> Thrust Control/1
  Sum1/1 -> PID Controller4/1
  Sum2/1 -> PID Controller5/1
  Sum/1 -> PID Controller3/1
  Bus Selector/1 -> Plot/2, Demux/1  "<Reference Velocity>"
  Reference Parameters/1 -> Bus Selector/1
  Bus Selector1/1 -> Plot/1, Demux1/1  "<Filtered Velocity>"
  Actual Parameters/1 -> Bus Selector1/1

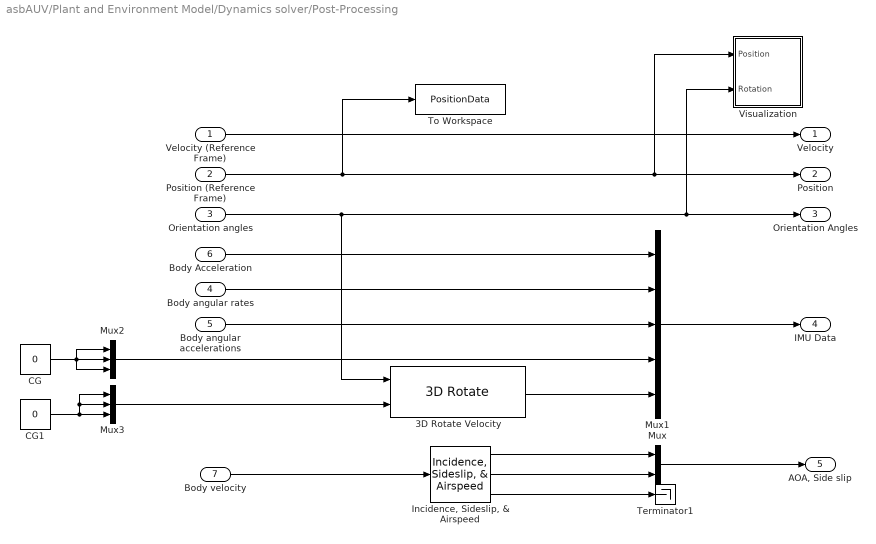
== system asbAUV/Plant and Environment Model/Dynamics solver/Post-Processing ==
  Velocity (Reference Frame) : Inport
  Position (Reference Frame) : Inport  Port=2
  Orientation angles : Inport  Port=3
  Body angular rates : Inport  Port=4
  Body angular accelerations : Inport  Port=5
  Body Acceleration : Inport  Port=6
  Body velocity : Inport  Port=7
  3D Rotate Velocity : asbAUVlib/3D Rotate   SystemSampleTime=-1  VariantActivationTime=update diagram  AllowFlexibleInterface=on  Latency=0  AutoFrameSizeCalculation=off
  CG : Constant  Value=0
  CG1 : Constant  Value=0
  "Incidence, Sideslip, & Airspeed" : aerolibasang/Incidence, Sideslip, & Airspeed
  Mux : Mux  Inputs=2
  Mux1 : Mux  Inputs=5
  Mux2 : Mux  Inputs=3
  Mux3 : Mux  Inputs=3
  Terminator1 : Terminator
  To Workspace : ToWorkspace  VariableName=PositionData  SampleTime=-1
  Visualization : Subsystem  mask(6DoF_Animation){u2=0.1, u8=on}
      mask prompts: u2 "aeroblks:aeroblkanim6dof:block6DoF_AnimationParamTimeintervalbetweenupdates"; u8 "aeroblks:aeroblkanim6dof:block6DoF_AnimationParamEnableanimation"
      mask help: aeroblks:aeroblkanim6dof:block6DoF_AnimationDesc
      mask init:
      | aeroicon('aeroblk');
      | Config.update = u2;
      | Config.Animenable = u8;
      | Config.Model = bdroot(gcb);
      mask Help: eval('asbhelp(''sixdof_animation'')');
      mask DialogControl DescGroupVar Prompt: Animation
      mask DialogControl DescTextVar Prompt: Show animation of body
      mask DialogControl u2 Prompt: Time interval between updates:
      mask DialogControl u8 Prompt: Enable animation
      mask Display:
      | port_label('input',1,'x_e','texmode','on');
      | port_label('input',2,'\phi \theta \psi','texmode','on');
  Velocity : Outport  VectorParamsAs1DForOutWhenUnconnected=off
  " Position" : Outport  Port=2  VectorParamsAs1DForOutWhenUnconnected=off
  Orientation Angles : Outport  Port=3  VectorParamsAs1DForOutWhenUnconnected=off
  IMU Data : Outport  Port=4  VectorParamsAs1DForOutWhenUnconnected=off
  "AOA, Side slip" : Outport  Port=5  VectorParamsAs1DForOutWhenUnconnected=off
  wires:
  Body angular accelerations/1 -> Mux1/3
  "Incidence, Sideslip, & Airspeed"/2 -> Mux/2
  Body velocity/1 -> "Incidence, Sideslip, & Airspeed"/1
  "Incidence, Sideslip, & Airspeed"/1 -> Mux/1
  Body angular rates/1 -> Mux1/2
  CG/1 -> Mux2/2, Mux2/1, Mux2/3
  3D Rotate Velocity/1 -> Mux1/5
  Mux2/1 -> Mux1/4
  Mux/1 -> "AOA, Side slip"/1
  CG1/1 -> Mux3/2, Mux3/1, Mux3/3
  Mux3/1 -> 3D Rotate Velocity/2
  Body Acceleration/1 -> Mux1/1
  Velocity (Reference Frame)/1 -> Velocity/1
  Orientation angles/1 -> 3D Rotate Velocity/1, Visualization/2(Rotation), Orientation Angles/1
  Mux1/1 -> IMU Data/1
  "Incidence, Sideslip, & Airspeed"/3 -> Terminator1/1
  Position (Reference Frame)/1 -> " Position"/1, Visualization/1(Position), To Workspace/1

== system asbAUV/Plant and Environment Model/Environmental Forces & Moments/Hydrodynamic Forces ==
  "Submarine Velocity (Body Axis) " : Inport
  "AOA, Side Slip" : Inport  Port=2
  Hydrodynamic Forces - Accurate : Subsystem  VariantControl=b==1
  Hydrodynamic Forces - Basic : Subsystem  VariantControl=b==0
  "Force due to Lift, Drag" : Outport  VectorParamsAs1DForOutWhenUnconnected=off

== system asbAUV/Plant and Environment Model/Environmental Forces & Moments/Hydrostatic Forces ==
  In1 : Inport
  Constant : Constant
  Environment Model : Subsystem  mask{ro=997, V=0.01, M=10, a=0, b=0, c=0}
      mask prompts: ro "Density of Water"; V "Volume of Submarine"; M "Mass of Submarine"; a "X Distance between CG and CB"; b "Y Distance between CG and CB"; c "Z Distance between CG and CB"
      mask DialogControl DescTextVar Prompt: Enter the Submarine related Parameters
      mask DialogControl Container3 Prompt: Distance between CG and Center of Buoyancy
  Hydrostatic Force : Outport  VectorParamsAs1DForOutWhenUnconnected=off
  Hydrostatic Moment : Outport  Port=2  VectorParamsAs1DForOutWhenUnconnected=off
  wires:
  Constant/1 -> Environment Model/1("Fraction submerged ")
  Environment Model/2(Moment due to Weight and Buoyancy) -> Hydrostatic Moment/1
  Environment Model/1(Forces due to Weight and Buoyancy) -> Hydrostatic Force/1
  In1/1 -> Environment Model/2(Orientation Angles)

== system asbAUV/Plant and Environment Model/Propulsion Forces & Moments/Force and moments due to Thrust ==
  Thrust Inputs : Inport
  "Thrust to Propulsion " : Subsystem
  Propulsion Force : Outport  VectorParamsAs1DForOutWhenUnconnected=off
  Propulsion Moment : Outport  Port=2  VectorParamsAs1DForOutWhenUnconnected=off
  wires:
  "Thrust to Propulsion "/2(Propulsion Moment) -> Propulsion Moment/1
  Thrust Inputs/1 -> "Thrust to Propulsion "/1(Thrust Inputs)
  "Thrust to Propulsion "/1(Propulsion Force) -> Propulsion Force/1

== system asbAUV/Plant and Environment Model/Propulsion Forces & Moments/Input commands to Thrust ==
  Thrust Control Inputs : Inport
  Demux : Demux  Outputs=3
  Input Commands to PWM : Subsystem
  "PWM Signals to Thrust " : Subsystem
  Thrust values : Outport  VectorParamsAs1DForOutWhenUnconnected=off
  wires:
  Input Commands to PWM/1(Px1) -> "PWM Signals to Thrust "/1(PWM Signal Px1)
  Input Commands to PWM/3(Py1) -> "PWM Signals to Thrust "/3(PWM Signal Py1)
  Demux/1 -> Input Commands to PWM/1(X Thruster)  "X Thrust Input"
  Demux/3 -> Input Commands to PWM/3(Z Thruster)  "Z Thrust Input"
  Input Commands to PWM/4(Py2) -> "PWM Signals to Thrust "/4(PWM Signal Py2)
  Demux/2 -> Input Commands to PWM/2(Y Thruster)  "Y Thrust Input"
  Input Commands to PWM/2(Px2) -> "PWM Signals to Thrust "/2(PWM Signal Px2)
  Input Commands to PWM/5(Pz) -> "PWM Signals to Thrust "/5(PWM Signal Pz)
  "PWM Signals to Thrust "/1(Thrust (N)) -> Thrust values/1
  Thrust Control Inputs/1 -> Demux/1

== system asbAUV/Sensor data and State Estimation/System With Noise/ Sensor (IMU) ==
  IMU Inputs : Inport
  Bus Creator : BusCreator  Inputs=2
  Bus Selector : BusSelector  OutputSignals=IMU Data
  Demux : Demux  Outputs=5
  Three-axis Inertial Measurement Unit : aerolibnav/Three-axis Inertial Measurement Unit  units=Metric (MKS)  imu=[0 0 0]  i_Ts=0  dtype_a=on  w_a=190  z_a=0.707  a_sf_cc=[1 0 0; 0 1 0; 0 0 1]  a_bias=[0 0 0]  a_sat="[-inf  -inf  -inf  inf inf inf]"  dtype_g=on  w_g=190  z_g=0.707  g_sf_cc=[1 0 0; 0 1 0; 0 0 1]  g_bias=[0 0 0]  g_sens=[0 0 0]  g_sat="[-inf  -inf  -inf  inf inf inf]"  i_rand=on  i_seeds=[23093 23094 23095 23096 23097 23098]  i_pow=[0.00001 0.00001 0.00001 0.00001 0.00001 0.00001]
  IMU Measurements : Outport  VectorParamsAs1DForOutWhenUnconnected=off
  wires:
  Three-axis Inertial Measurement Unit/1 -> Bus Creator/1  "IMU Measured Acceleration"
  Demux/2 -> Three-axis Inertial Measurement Unit/2
  Demux/4 -> Three-axis Inertial Measurement Unit/4
  Demux/5 -> Three-axis Inertial Measurement Unit/5
  Demux/3 -> Three-axis Inertial Measurement Unit/3
  Demux/1 -> Three-axis Inertial Measurement Unit/1
  Three-axis Inertial Measurement Unit/2 -> Bus Creator/2  "IMU Measured Body Rates"
  IMU Inputs/1 -> Bus Selector/1
  Bus Selector/1 -> Demux/1  "<IMU Data>"
  Bus Creator/1 -> IMU Measurements/1

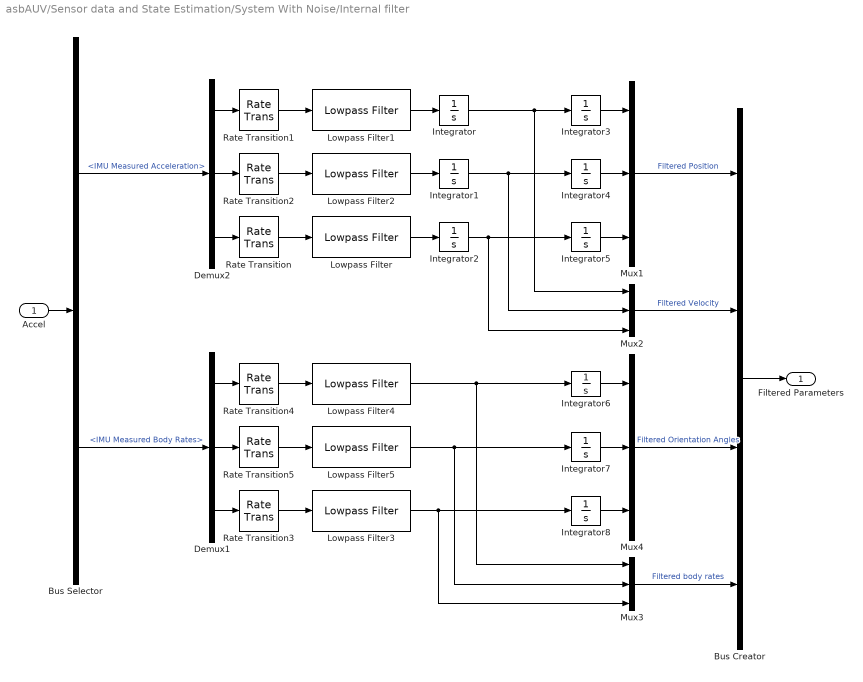
== system asbAUV/Sensor data and State Estimation/System With Noise/Internal filter ==
  Accel : Inport
  Bus Creator : BusCreator  Inputs=4
  Bus Selector : BusSelector  OutputSignals=IMU Measured Acceleration,IMU Measured Body Rates
  Demux1 : Demux  Outputs=3
  Demux2 : Demux  Outputs=3
  Integrator{,1..8} (9 alike) : Integrator
  Lowpass Filter{,1..5} (6 alike) : dspfdesign/Lowpass Filter  FilterType=FIR  DesignForMinimumOrder=on  FilterOrder=50  PassbandFrequency=1/100  StopbandFrequency=45  PassbandRipple=0.1  StopbandAttenuation=80  SampleRateMode=Specify on dialog  SampleRate=100  SimulateUsing=Interpreted execution  roundingMode=Floor  coeffsDataTypeStr=fixdt(1,16)
  Mux{1..4} (4 alike) : Mux  Inputs=3
  Rate Transition{,1..5} (6 alike) : RateTransition  OutPortSampleTime=0.01
  Filtered Parameters : Outport  VectorParamsAs1DForOutWhenUnconnected=off
  wires:
  Rate Transition5/1 -> Lowpass Filter5/1
  Rate Transition4/1 -> Lowpass Filter4/1
  Demux1/1 -> Rate Transition4/1
  Lowpass Filter3/1 -> Integrator8/1, Mux3/3
  Demux1/2 -> Rate Transition5/1
  Lowpass Filter5/1 -> Integrator7/1, Mux3/2
  Lowpass Filter4/1 -> Integrator6/1, Mux3/1
  Integrator6/1 -> Mux4/1
  Rate Transition3/1 -> Lowpass Filter3/1
  Integrator8/1 -> Mux4/3
  Demux1/3 -> Rate Transition3/1
  Integrator7/1 -> Mux4/2
  Accel/1 -> Bus Selector/1
  Bus Selector/1 -> Demux2/1  "<IMU Measured Acceleration>"
  Bus Selector/2 -> Demux1/1  "<IMU Measured Body Rates>"
  Mux4/1 -> Bus Creator/3  "Filtered Orientation Angles"
  Mux3/1 -> Bus Creator/4  "Filtered body rates"
  Bus Creator/1 -> Filtered Parameters/1
  Integrator2/1 -> Integrator5/1, Mux2/3
  Integrator/1 -> Integrator3/1, Mux2/1
  Mux2/1 -> Bus Creator/2  "Filtered Velocity"
  Mux1/1 -> Bus Creator/1  "Filtered Position"
  Lowpass Filter/1 -> Integrator2/1
  Demux2/2 -> Rate Transition2/1
  Rate Transition1/1 -> Lowpass Filter1/1
  Integrator4/1 -> Mux1/2
  Demux2/3 -> Rate Transition/1
  Lowpass Filter2/1 -> Integrator1/1
  Lowpass Filter1/1 -> Integrator/1
  Demux2/1 -> Rate Transition1/1
  Integrator5/1 -> Mux1/3
  Integrator1/1 -> Integrator4/1, Mux2/2
  Rate Transition/1 -> Lowpass Filter/1
  Integrator3/1 -> Mux1/1
  Rate Transition2/1 -> Lowpass Filter2/1

== system asbAUV/Plant and Environment Model/Dynamics solver/Post-Processing/Visualization ==
  Position : Inport
  Rotation : Inport  Port=2  Unit=rad
  Animation S-Function : M-S-Function  FunctionName=asbAUVax  Parameters=Config
  Mux4 : Mux  Inputs=2
  wires:
  Rotation/1 -> Mux4/2
  Mux4/1 -> Animation S-Function/1
  Position/1 -> Mux4/1

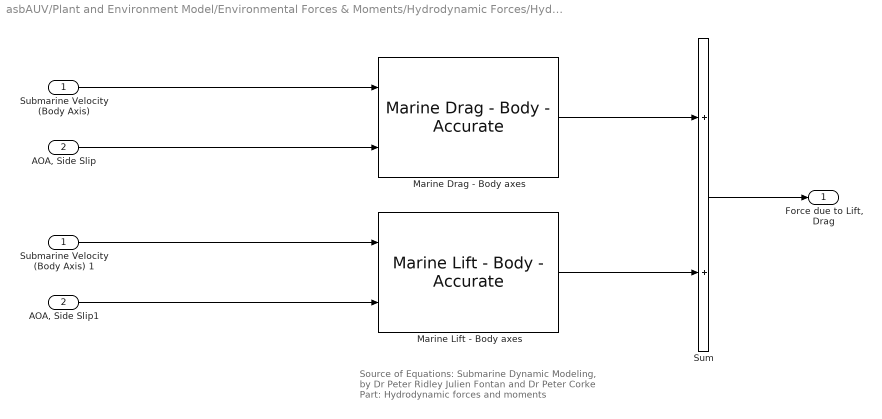
== system asbAUV/Plant and Environment Model/Environmental Forces & Moments/Hydrodynamic Forces/Hydrodynamic Forces - Accurate ==
  note: Source of Equations:
      | Submarine Dynamic Modeling, by
      | Dr Peter Ridley Julien Fontan and Dr Peter Corke
      |
      | Part: Hydrodynamic forces and moments
  "Submarine Velocity (Body Axis) " : Inport
  "AOA, Side Slip" : Inport  Port=2
  "AOA, Side Slip1" : InportShadow  Port=2
  Marine Drag - Body axes : asbAUVlib/Marine Drag - Body - Accurate  SystemSampleTime=-1  VariantActivationTime=update diagram  AllowFlexibleInterface=on  Latency=0  AutoFrameSizeCalculation=off
  Marine Lift - Body axes : asbAUVlib/Marine Lift - Body - Accurate  SystemSampleTime=-1  VariantActivationTime=update diagram  AllowFlexibleInterface=on  Latency=0  AutoFrameSizeCalculation=off
  Submarine Velocity (Body Axis) 1 : InportShadow
  Sum : Sum
  "Force due to Lift, Drag" : Outport  VectorParamsAs1DForOutWhenUnconnected=off
  wires:
  Marine Drag - Body axes/1 -> Sum/1
  Marine Lift - Body axes/1 -> Sum/2
  "AOA, Side Slip"/1 -> Marine Drag - Body axes/2
  "Submarine Velocity (Body Axis) "/1 -> Marine Drag - Body axes/1
  Sum/1 -> "Force due to Lift, Drag"/1
  "AOA, Side Slip1"/1 -> Marine Lift - Body axes/2
  Submarine Velocity (Body Axis) 1/1 -> Marine Lift - Body axes/1

== system asbAUV/Plant and Environment Model/Environmental Forces & Moments/Hydrodynamic Forces/Hydrodynamic Forces - Basic ==
  "Submarine Velocity (Body Axis) " : Inport
  "AOA, Side Slip" : Inport  Port=2
  "AOA, Side Slip1" : InportShadow  Port=2
  Marine Drag - Body Axes : asbAUVlib/Marine Drag - Body - Approximate  SystemSampleTime=-1  VariantActivationTime=update diagram  AllowFlexibleInterface=on  Latency=0  AutoFrameSizeCalculation=off
  Marine Lift - Body Axes : asbAUVlib/Marine Lift - Body - Approximate  SystemSampleTime=-1  VariantActivationTime=update diagram  AllowFlexibleInterface=on  Latency=0  AutoFrameSizeCalculation=off
  Submarine Velocity (Body Axis) 1 : InportShadow
  Sum : Sum
  "Force due to Lift, Drag" : Outport  VectorParamsAs1DForOutWhenUnconnected=off
  wires:
  Marine Drag - Body Axes/1 -> Sum/1
  Marine Lift - Body Axes/1 -> Sum/2
  "AOA, Side Slip"/1 -> Marine Lift - Body Axes/2
  "Submarine Velocity (Body Axis) "/1 -> Marine Drag - Body Axes/1
  Sum/1 -> "Force due to Lift, Drag"/1
  "AOA, Side Slip1"/1 -> Marine Drag - Body Axes/2
  Submarine Velocity (Body Axis) 1/1 -> Marine Lift - Body Axes/1

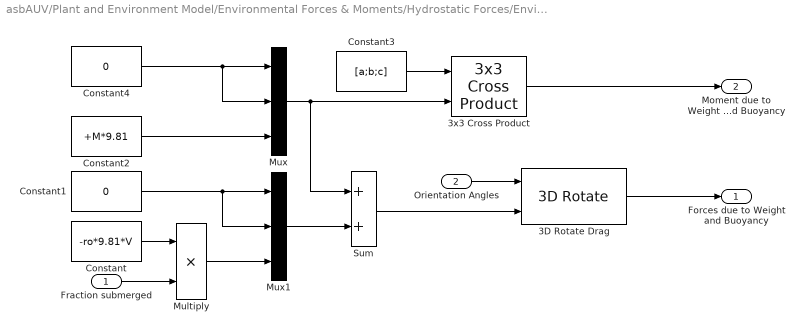
== system asbAUV/Plant and Environment Model/Environmental Forces & Moments/Hydrostatic Forces/Environment Model ==
  "Fraction submerged " : Inport
  Orientation Angles : Inport  Port=2
  3D Rotate Drag : asbAUVlib/3D Rotate   SystemSampleTime=-1  VariantActivationTime=update diagram  AllowFlexibleInterface=on  Latency=0  AutoFrameSizeCalculation=off
  3x3 Cross Product : sharedutil/3x3 Cross Product  aMode=aMode
      settings: LibrarySourceBlock=aerolibutil/3x3 Cross Product
  Constant : Constant  Value=-ro*9.81*V
  Constant1 : Constant  Value=0
  Constant2 : Constant  Value=+M*9.81
  Constant3 : Constant  Value=[a;b;c]
  Constant4 : Constant  Value=0
  Multiply : Product
  Mux : Mux  Inputs=3
  Mux1 : Mux  Inputs=3
  Sum : Sum
  Forces due to Weight and Buoyancy : Outport  VectorParamsAs1DForOutWhenUnconnected=off
  Moment due to Weight and Buoyancy : Outport  Port=2  VectorParamsAs1DForOutWhenUnconnected=off
  wires:
  3x3 Cross Product/1 -> Moment due to Weight and Buoyancy/1
  Constant3/1 -> 3x3 Cross Product/1
  "Fraction submerged "/1 -> Multiply/2
  Mux1/1 -> Sum/2
  Multiply/1 -> Mux1/3
  Mux/1 -> 3x3 Cross Product/2, Sum/1
  Constant/1 -> Multiply/1
  Constant1/1 -> Mux1/2, Mux1/1
  Constant2/1 -> Mux/3
  Sum/1 -> 3D Rotate Drag/2
  Orientation Angles/1 -> 3D Rotate Drag/1
  3D Rotate Drag/1 -> Forces due to Weight and Buoyancy/1
  Constant4/1 -> Mux/1, Mux/2

== system asbAUV/Plant and Environment Model/Propulsion Forces & Moments/Force and moments due to Thrust/Thrust to Propulsion  ==
  Thrust Inputs : Inport
  Demux : Demux  Outputs=5
  Moment computation : Subsystem
  Sum : Sum  Inputs=+++++
  Thrust Transformation : Subsystem
  Propulsion Force : Outport  VectorParamsAs1DForOutWhenUnconnected=off
  Propulsion Moment : Outport  Port=2  VectorParamsAs1DForOutWhenUnconnected=off
  wires:
  Demux/5 -> Moment computation/5(Pz)
  Demux/4 -> Moment computation/4(Py2)
  Demux/3 -> Moment computation/3(Py1)
  Demux/2 -> Moment computation/2(Px2)
  Demux/1 -> Moment computation/1(Px1)
  Thrust Transformation/3(Thrust Py1) -> Sum/3
  Moment computation/1(Moment) -> Propulsion Moment/1
  Thrust Transformation/4(Thrust Py2) -> Sum/4
  Thrust Transformation/5(Thrust Pz) -> Sum/5
  Sum/1 -> Propulsion Force/1
  Thrust Inputs/1 -> Thrust Transformation/1(Thrust Inputs), Demux/1
  Thrust Transformation/1(Thrust Px1) -> Sum/1
  Thrust Transformation/2(Thrust Px2) -> Sum/2

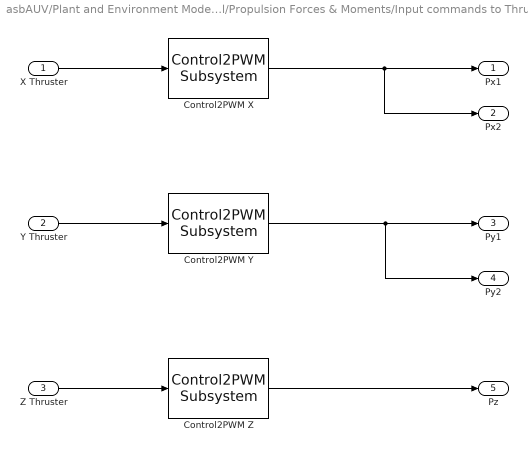
== system asbAUV/Plant and Environment Model/Propulsion Forces & Moments/Input commands to Thrust/Input Commands to PWM ==
  X Thruster : Inport
  Y Thruster : Inport  Port=2
  Z Thruster : Inport  Port=3
  Control2PWM X : asbAUVlib/Control2PWM Subsystem  SystemSampleTime=-1  VariantActivationTime=update diagram  AllowFlexibleInterface=on  Latency=0  AutoFrameSizeCalculation=off
  Control2PWM Y : asbAUVlib/Control2PWM Subsystem  SystemSampleTime=-1  VariantActivationTime=update diagram  AllowFlexibleInterface=on  Latency=0  AutoFrameSizeCalculation=off
  Control2PWM Z : asbAUVlib/Control2PWM Subsystem  SystemSampleTime=-1  VariantActivationTime=update diagram  AllowFlexibleInterface=on  Latency=0  AutoFrameSizeCalculation=off
  Px1 : Outport  VectorParamsAs1DForOutWhenUnconnected=off
  Px2 : Outport  Port=2  VectorParamsAs1DForOutWhenUnconnected=off
  Py1 : Outport  Port=3  VectorParamsAs1DForOutWhenUnconnected=off
  Py2 : Outport  Port=4  VectorParamsAs1DForOutWhenUnconnected=off
  Pz : Outport  Port=5  VectorParamsAs1DForOutWhenUnconnected=off
  wires:
  Control2PWM Z/1 -> Pz/1
  Y Thruster/1 -> Control2PWM Y/1
  Control2PWM Y/1 -> Py1/1, Py2/1
  Z Thruster/1 -> Control2PWM Z/1
  Control2PWM X/1 -> Px1/1, Px2/1
  X Thruster/1 -> Control2PWM X/1
